simulink model "SIM_LIN"  (R2024b)
settings: Solver=VariableStepAuto  StartTime=0.0  StopTime=30  RelTol=1e-3
values from neighbouring files (symbols this model uses):
  Anom = A.NominalValue    [Parameter_CSI.m]
  Bnom = B.NominalValue    [Parameter_CSI.m]
  C = [(b_true*(R_rear/L)^2-a_true*(R_rear^2))*phi_dot*psi_dot*sin(psi)*cos(psi)+c_phi*phi_dot; -Ipz*(R_rear/L)*phi_dot*psi_dot*cos(psi)+c_psi*psi_dot]    [Dynamics_CSI.m]    (also in Parameter_CSI.m = [1 0 0 0 0;0 0 1 0 0])
  D = append(d1,d1,tf(eye(2)),tf(eye(2)))    [D_K_controller2_FINAL.m]    (also in Parameter_CSI.m = zeros(2,2))
  u_eq = [c_phi*vx/R_rear_nom; 0]    [Parameter_CSI.m]
  x_eq = [0; 0; vx/R_rear_nom; 0; 0]    [Parameter_CSI.m]
settings Model: Creator=alebe  LastModifiedBy=rober

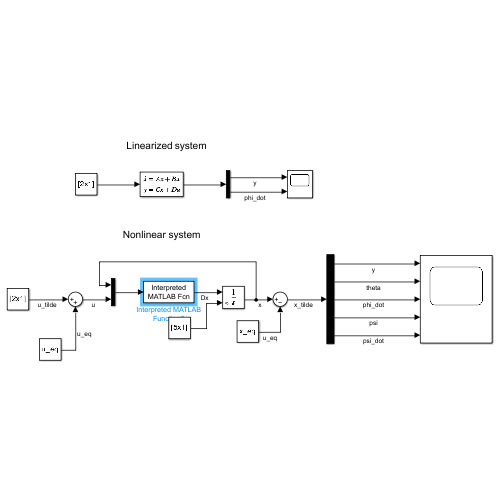
[thumbnail: Simulink's stored preview of the top-level diagram]
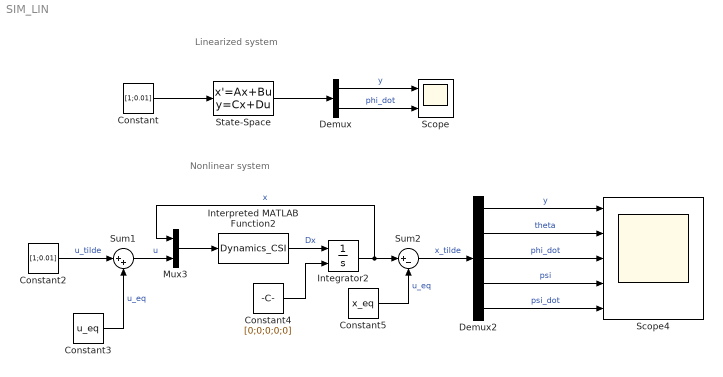
== system SIM_LIN ==
  note: Linearized system
  note: Nonlinear system
  Constant : Constant  Value=[1;0.01]
  Constant2 : Constant  Value=[1;0.01]
  Constant3 : Constant  Value=u_eq
  Constant4 : Constant  Value=[0;0;0;0;0]
  Constant5 : Constant  Value=x_eq
  Demux : Demux  Outputs=2
  Demux2 : Demux  Outputs=5
  Integrator2 : Integrator  InitialConditionSource=external
  Interpreted MATLAB Function2 : MATLABFcn  MATLABFcn=Dynamics_CSI
  Mux3 : Mux  Inputs=2
  Scope : Scope  NumInputPorts=2
  Scope4 : Scope  NumInputPorts=5
  State-Space : StateSpace  A=Anom  B=Bnom  C=C  D=D  InitialCondition=0
  Sum1 : Sum  Inputs=|++
  Sum2 : Sum  Inputs=|+-
  wires:
  State-Space/1 -> Demux/1
  Demux/1 -> Scope/1  "y"
  Demux/2 -> Scope/2  "phi_dot"
  Constant/1 -> State-Space/1
  Constant2/1 -> Sum1/1  "u_tilde"
  Constant3/1 -> Sum1/2  "u_eq"
  Sum2/1 -> Demux2/1  "x_tilde"
  Demux2/1 -> Scope4/1  "y"
  Mux3/1 -> Interpreted MATLAB Function2/1
  Demux2/2 -> Scope4/2  "theta"
  Demux2/3 -> Scope4/3  "phi_dot"
  Demux2/5 -> Scope4/5  "psi_dot"
  Interpreted MATLAB Function2/1 -> Integrator2/1  "Dx"
  Sum1/1 -> Mux3/2  "u"
  Demux2/4 -> Scope4/4  "psi"
  Constant5/1 -> Sum2/2  "u_eq"
  Integrator2/1 -> Mux3/1, Sum2/1  "x"
  Constant4/1 -> Integrator2/2
